simulink subsystem "AudioRecive"  (R2024b)
settings: Solver=VariableStepAuto  StartTime=0.0  StopTime=10.0  RelTol=1e-3
undefined symbols (not defined in the file or in its folder): Param
libraries: dspsnks4 x1, simulink x1, dspquant2 x1
settings Model: Creator=fredr  LastModifiedBy=fredr

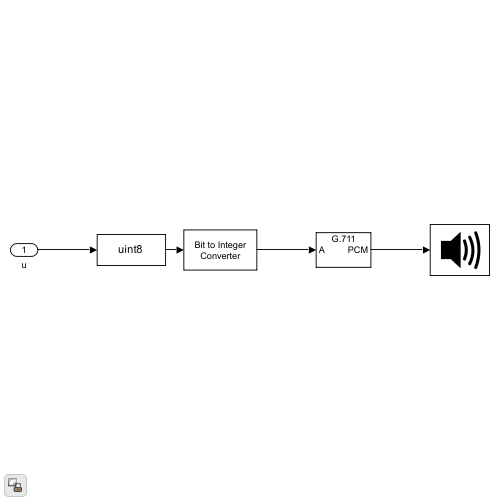
[thumbnail: Simulink's stored preview of the top-level diagram]
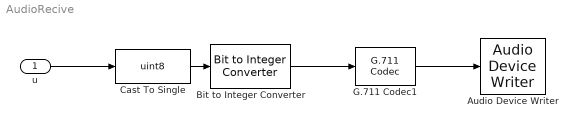
== system AudioRecive ==
  u : Inport
  Audio Device Writer : dspsnks4/Audio Device Writer  Driver=DirectSound  Device=Default  InheritSampleRate=off  SampleRate=200/Param.FrameTime  BitDepth=16-bit integer  BufferSize=4096  NumBuffers=10  DefaultOutputChannelMapping=on  OutputChannelMapping=1:2  OutputNumUnderrunSamples=off  DriverIdx=1  DeviceWarnFlag=''
  Bit to Integer Converter : simulink/Logic and Bit Operations/Bit to Integer Converter  nbits=8  bitOrder=MSB first  signedOutputValues=Unsigned  outDtype=Inherit via internal rule  outDtypeSigned=Inherit via internal rule
  Cast To Single : DataTypeConversion  OutDataTypeStr=uint8  SaturateOnIntegerOverflow=off  RndMeth=Floor
  G.711 Codec1 : dspquant2/G.711 Codec  mode=Decode A-law to PCM  errmode=Warning
  wires:
  u/1 -> Cast To Single/1
  Bit to Integer Converter/1 -> G.711 Codec1/1
  G.711 Codec1/1 -> Audio Device Writer/1
  Cast To Single/1 -> Bit to Integer Converter/1
